simulink model "q4"  (R2020b)
settings: Solver=VariableStepAuto  StartTime=0.0  StopTime=10.0  MaxStep=0.001  RelTol=1e-3
settings Model: Creator=Ravi  LastModifiedBy=Ravi

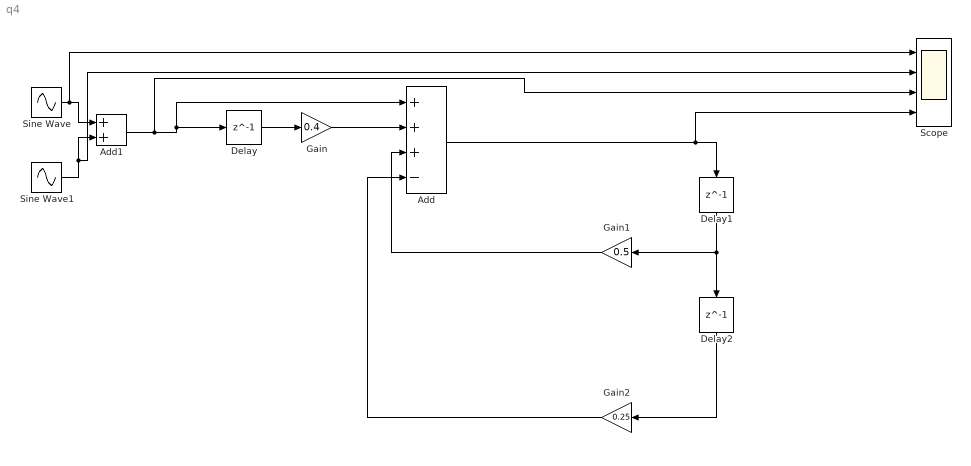
== system q4 ==
  Add : Sum  Inputs=+++-
  Add1 : Sum
  Delay : Delay  DelayLength=1
  Delay1 : Delay  DelayLength=1
  Delay2 : Delay  DelayLength=1
  Gain : Gain  Gain=0.4
  Gain1 : Gain  Gain=0.5
  Gain2 : Gain  Gain=0.25
  Scope : Scope  NumInputPorts=4
  Sine Wave : Sin  SampleTime=0
  Sine Wave1 : Sin  Amplitude=0.5  Frequency=50  SampleTime=0
  wires:
  Delay/1 -> Gain/1
  Gain/1 -> Add/2
  Add/1 -> Scope/4, Delay1/1
  Delay1/1 -> Gain1/1, Delay2/1
  Delay2/1 -> Gain2/1
  Gain1/1 -> Add/3
  Gain2/1 -> Add/4
  Sine Wave/1 -> Scope/1, Add1/1
  Sine Wave1/1 -> Scope/2, Add1/2
  Add1/1 -> Scope/3, Delay/1, Add/1
